simulink model "controller_model"  (R2020b)
settings: Solver=VariableStepAuto  StartTime=0.0  StopTime=10.0  RelTol=1e-3
settings Model: Creator=fion  LastModifiedBy=fion

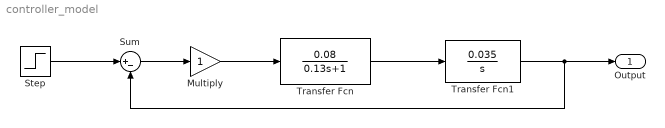
== system controller_model ==
  Multiply : Gain
  Step : Step  SampleTime=0
  Sum : Sum  Inputs=|+-
  Transfer Fcn : TransferFcn  Numerator=[0.08]  Denominator=[0.13 1]
  Transfer Fcn1 : TransferFcn  Numerator=[0.035]  Denominator=[1 0]
  Output : Outport
  wires:
  Transfer Fcn/1 -> Transfer Fcn1/1
  Multiply/1 -> Transfer Fcn/1
  Step/1 -> Sum/1
  Sum/1 -> Multiply/1
  Transfer Fcn1/1 -> Output/1, Sum/2
